simulink library "engine_JetCatP120SE_lib"  (Simulink 6.6)
libraries: simulink x5
settings Model: Creator=amurch  LastModifiedBy=amurch

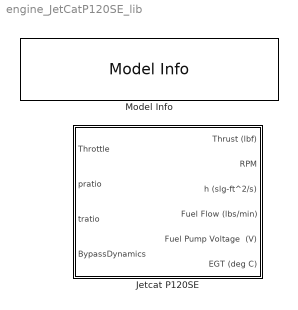
== system engine_JetCatP120SE_lib ==
  Jetcat P120SE : Subsystem
      mask init:
      | % Curve fit parameters for Jetcat P120SE Model
      | Coeff_thrust   = [ 3E-5  -0.0011  0.0868  -1.1447];
      | Coeff_throttle = [4E-5 -0.0098 1.2879 27.906];
      | Coeff_fuelflow = [4E-5 0.0037, 0.0345];
      | Coeff_tau      = [ -2.2400e-02   2.9948e+00];
      | Coeff_EGT      = [ 2E-5, -0.0036,0.2342,-8.0496,664.99]; %EGT model, deg C
      | fuelpump_table = [0 0.576	0.625	0.6985	0.7845	0.8575	0.919	0.9805	1.0415	1.1025...
      |                     1.1515	1.262	1.287	1.373	1.52	1.618	1.74	1.887	1.973...
      |                     2.12	2.255	2.4385	2.647	2.7575	2.9905	3.162]; %volts, table of fuel pump voltages
      | fuelflow_table = [0,0.0794,0.0876,0.102,0.1149,0.1275,0.1379,0.1487,0.1586,0.1671,...
      |                     0.1775,0.1858,0.194,0.2038,0.2206,0.2405,0.2566,0.2746,0.2921,0.3102,...
      |                     0.3266,0.3445,0.3533,0.3611,0.3866,0.4083;]*2; %lbs/min,   FULL fuel flow rates corresponding to pump voltages (fuelpump_table)  
      | % Equvalent Shaft parameters for engine
      | shaft_dia = 0.75/12.0;       % diameter of rotating turbine in feet 
      | shaft_len = 6.25/12.0;       % length of rotating turbine in feet   
      | density   = 15.2;            % mass density of steel in slugs/ft^3
  Model Info : simulink/Model-Wide Utilities/Model Info  SystemSampleTime=-1  InitialBlockCM=None  BlockCM=None  Frame=on  DisplayStringWithTags=|  HorizontalTextAlignment=Center  LeftAlignmentValue=0.5  SourceBlockDiagram=engine_JetCatP120SE_lib  TagMaxNumber=20
      | JetCat P120SE Engine Library
      | 
      | Model Version: %<ModelVersion>
      | Last modifed by %<LastModifiedBy> on %<LastModificationDate>

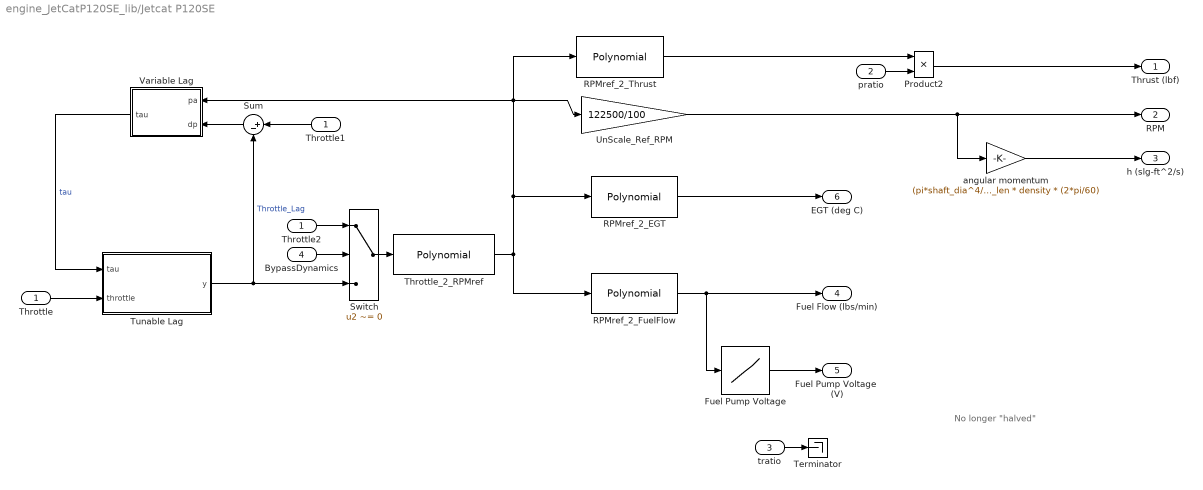
== system engine_JetCatP120SE_lib/Jetcat P120SE ==
  note: No longer "halved"
  Throttle : Inport
  pratio : Inport  Port=2
  tratio : Inport  Port=3
  BypassDynamics : Inport  Port=4
  Fuel Pump Voltage : Lookup  InputValues=fuelflow_table  OutputValues=fuelpump_table  LookUpMeth=Interpolation-Use End Values
  Product2 : Product  RndMeth=Zero
  RPMref_2_EGT : simulink/Math Operations/Polynomial  coefs=Coeff_EGT
  RPMref_2_FuelFlow : simulink/Math Operations/Polynomial  coefs=Coeff_fuelflow
  RPMref_2_Thrust : simulink/Math Operations/Polynomial  coefs=Coeff_thrust
  Sum : Sum  Orientation=left  Inputs=|+-
  Switch : Switch  Criteria=u2 ~= 0
  Terminator : Terminator
  Throttle1 : InportShadow  Orientation=left  Port=1  LatchByCopyingInsideSignal=off
  Throttle2 : InportShadow  Port=1  LatchByCopyingInsideSignal=off
  Throttle_2_RPMref : simulink/Math Operations/Polynomial  coefs=Coeff_throttle
  Tunable Lag : Subsystem
  UnScale_Ref_RPM : Gain  Gain=122500/100
  Variable Lag : Stateflow chart  Orientation=left
  angular momentum : Gain  Gain=(pi*shaft_dia^4/32) * shaft_len * density * (2*pi/60)
  Thrust (lbf) : Outport
  RPM : Outport  Port=2
  h (slg-ft^2/s) : Outport  Port=3
  Fuel Flow (lbs/min) : Outport  Port=4
  Fuel Pump Voltage  (V) : Outport  Port=5
  EGT (deg C) : Outport  Port=6
  wires:
  Variable Lag/1(tau) -> Tunable Lag/1(tau)  "tau"
  Throttle/1 -> Tunable Lag/2(throttle)
  Tunable Lag/1(y) -> Sum/2, Switch/3  "Throttle_Lag"
  Throttle_2_RPMref/1 -> RPMref_2_FuelFlow/1, Variable Lag/1(pa), RPMref_2_Thrust/1, UnScale_Ref_RPM/1, RPMref_2_EGT/1
  angular momentum/1 -> h (slg-ft^2/s)/1
  UnScale_Ref_RPM/1 -> angular momentum/1, RPM/1
  tratio/1 -> Terminator/1
  RPMref_2_Thrust/1 -> Product2/1
  Product2/1 -> Thrust (lbf)/1
  RPMref_2_FuelFlow/1 -> Fuel Flow (lbs/min)/1, Fuel Pump Voltage/1
  pratio/1 -> Product2/2
  Fuel Pump Voltage/1 -> Fuel Pump Voltage  (V)/1
  RPMref_2_EGT/1 -> EGT (deg C)/1
  Sum/1 -> Variable Lag/2(dp)
  Throttle1/1 -> Sum/1
  BypassDynamics/1 -> Switch/2
  Throttle2/1 -> Switch/1
  Switch/1 -> Throttle_2_RPMref/1

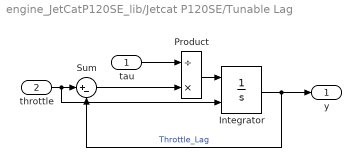
== system engine_JetCatP120SE_lib/Jetcat P120SE/Tunable Lag ==
  tau : Inport
  throttle : Inport  Port=2
  Integrator : Integrator  InitialConditionSource=external
  Product : Product  Inputs=/*  RndMeth=Zero
  Sum : Sum  Inputs=|+-
  y : Outport
  wires:
  throttle/1 -> Integrator/2, Sum/1
  tau/1 -> Product/1
  Sum/1 -> Product/2
  Product/1 -> Integrator/1
  Integrator/1 -> y/1, Sum/2  "Throttle_Lag"

== matlab function Jetcat P120SE/Variable Lag ==
  data: pa input inherited; dp input inherited; tau output inherited
function tau = fcn(pa,dp)
% This block supports an embeddable subset of the MATLAB language.
% See the help menu for details.


if dp >= 0
    if pa >= 50
        tau=1.44;  % time constant = 1.44 sec.
    else
        tau=1.96;  % time constant = 1.96 sec.
    end
else
    %
    %  Power decrease.
    %
    if pa >= 50
        tau=0.85;  % time constant = 0.85 sec.
    else
        tau=1.43;  % time constant = 1.43 sec.
    end
end
